simulink model "Hierarchy3"  (Simulink 8.7)
settings: Solver=ode45  StartTime=0.0  StopTime=10.0  RelTol=1e-3
settings Model: Creator=scaife  LastModifiedBy=bourbouh  ExtModeAutoUpdateStatusClock=off
settings DataIOCC: SignalLoggingSaveFormat=ModelDataLogs  SignalLoggingName=sigsOut
settings DebuggingCC: SaveWithParameterizedLinksMsg=none  SignalResolutionControl=TryResolveAllWithWarning  MultiTaskDSMMsg=warning  MultiTaskCondExecSysMsg=none
settings HardwareCC: TargetUnknown=on
settings SFSimCC: SimParseCustomCode=off
settings GRTTargetCC: GeneratePreprocessorConditionals=Use local settings  CombineOutputUpdateFcns=off  GRTInterface=on

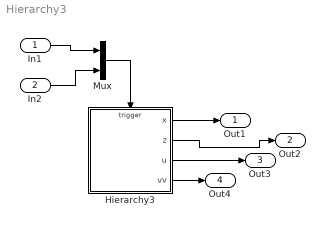
== system Hierarchy3 ==
  In1 : Inport
  In2 : Inport  Port=2
  Hierarchy3 : Stateflow chart  TreatAsAtomicUnit=on
  Mux : Mux  Inputs=2
  Out1 : Outport
  Out2 : Outport  Port=2
  Out3 : Outport  Port=3
  Out4 : Outport  Port=4
  wires:
  Hierarchy3/1(x) -> Out1/1
  Hierarchy3/2(z) -> Out2/1
  Hierarchy3/3(u) -> Out3/1
  Hierarchy3/4(vv) -> Out4/1
  In1/1 -> Mux/1
  In2/1 -> Mux/2
  Mux/1 -> Hierarchy3/Trigger

== stateflow chart Hierarchy3 ==
  state TOP1 [parallel]
    settings: executionOrder=1
    state A
      state A1/
        en: x=0
      state A2/
        en: x=5
      (junction 17) -> A1 [order 2]
      (default) -> A1
      A2 -> (junction 17) : E[x>0]{y=-1}
      (junction 17) -> (junction 18) [order 1] : [x<=5]{x+=y}
      (junction 18) -> (junction 17) [order 2] : {x+=y}
      A1 -> (junction 18) : E[x<5]{y=1}
      (junction 18) -> A2 [order 1] : [x>=5]
    state B
      state B1/
        en: z=0
      state B2/
        en: z=5
      (junction 26) -> B1 [order 2]
      (default) -> B1
      B2 -> (junction 26) : E[z>0]{y=-1}
      (junction 26) -> (junction 27) [order 1] : [z<=5]{z+=y}
      (junction 27) -> (junction 26) [order 2] : {z+=y}
      B1 -> (junction 27) : E[z<5]{y=1}
      (junction 27) -> B2 [order 1] : [z>=5]
    (default) -> A
    (junction 35) -> A [order 2]
    A -> (junction 36) : F{i=0}
    (junction 35) -> (junction 35) [order 1] : [i>0]{i--}
    B -> (junction 35) : F{i=3}
    (junction 36) -> (junction 36) [order 1] : [i<3]{i++}
    (junction 36) -> B [order 2]
  state TOP2 [parallel]
    settings: executionOrder=2
    state C
      state C1/
        en: vv=0
      state C2/
        en:vv=5
      (junction 53) -> C1 [order 2]
      (default) -> C1
      C2 -> (junction 53) : E[vv>0]{w=-1}
      (junction 53) -> (junction 54) [order 1] : [vv<=5]{vv+=w}
      (junction 54) -> (junction 53) [order 2] : {vv+=w}
      C1 -> (junction 54) : E[vv<5]{w=1}
      (junction 54) -> C2 [order 1] : [vv>=5]
    state D
      state D1/
        en: u=0
      state D2/
        en: u=5
      (junction 62) -> D1 [order 2]
      (default) -> D1
      D2 -> (junction 62) : E[u>0]{w=-1}
      (junction 62) -> (junction 63) [order 1] : [u<=5]{u+=w}
      (junction 63) -> (junction 62) [order 2] : {u+=w}
      D1 -> (junction 63) : E[u<5]{w=1}
      (junction 63) -> D2 [order 1] : [u>=5]
    (default) -> C
    (junction 44) -> C [order 2]
    C -> (junction 45) : F{j=0}
    (junction 44) -> (junction 44) [order 1] : [j>0]{j--}
    D -> (junction 44) : F{j=3}
    (junction 45) -> (junction 45) [order 1] : [j<3]{j++}
    (junction 45) -> D [order 2]
  data: y local int32; x output int32; z output int32; i local int32; j local int32; w local int32; u output int32; vv output int32
  events: E input EITHER_EDGE_EVENT; F input EITHER_EDGE_EVENT
